simulink model "parafoil_CMA"  (R2024a)
settings: Solver=ode4  StartTime=0.0  StopTime=500  FixedStep=2e-2  RelTol=1e-3
undefined symbols (not defined in the file): F, height_action, MIL, Severe
libraries: aerolibwind2 x1
settings Model: Creator=Long  LastModifiedBy=Yang
settings SolverCC: AlgebraicLoopSolver=TrustRegion
settings DebuggingCC: UnconnectedInputMsg=warning  UnconnectedOutputMsg=warning  UnconnectedLineMsg=warning
settings ModelReferenceCC: EnableRefExpFcnMdlSchedulingChecks=on
settings SFSimCC: CustomCodeUndefinedFunction=UseInterfaceOnly
settings RTWCC: GPUComputeCapability=3.5

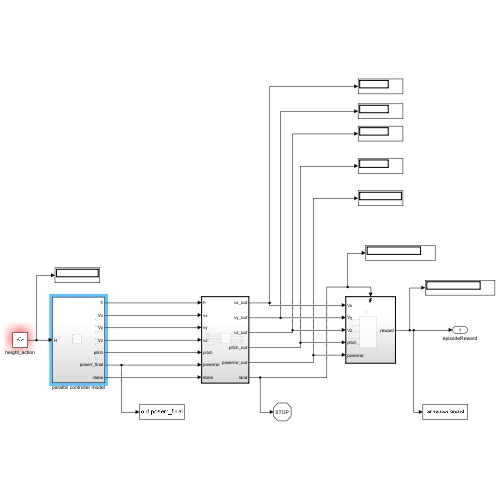
[thumbnail: Simulink's stored preview of the top-level diagram]
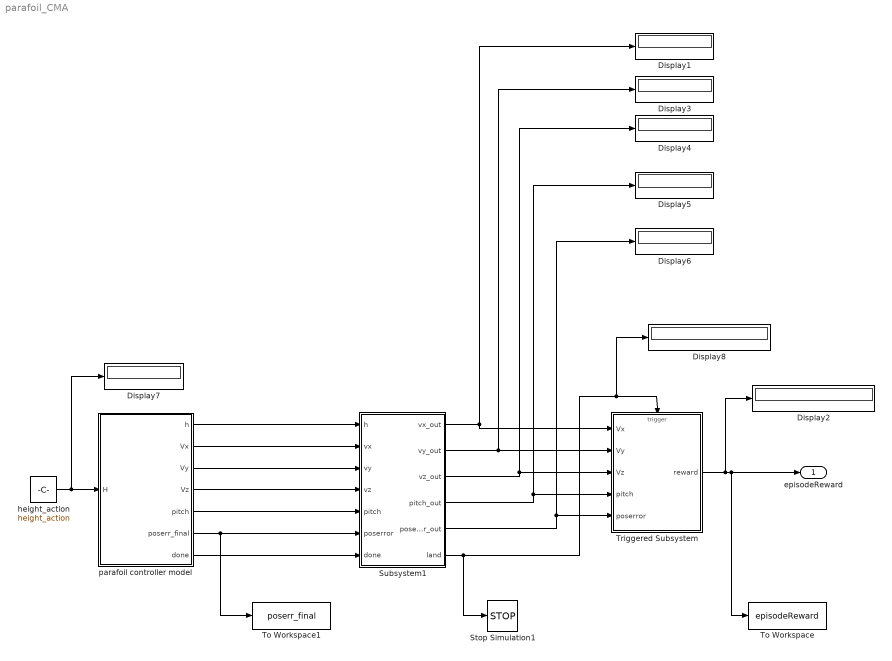
== system parafoil_CMA ==
  Display{1..8} (8 alike) : Display
  Stop Simulation1 : Stop
  Subsystem1 : Subsystem  TreatAsAtomicUnit=on  SystemSampleTime=0.02
  To Workspace : ToWorkspace  VariableName=episodeReward  SampleTime=-1
      settings: MaxDataPoints=1
  To Workspace1 : ToWorkspace  VariableName=poserr_final  SampleTime=-1
      settings: MaxDataPoints=1
  Triggered Subsystem : Subsystem  TreatAsAtomicUnit=on
  height_action : Constant  Value=height_action
  parafoil controller model : Subsystem
  episodeReward : Outport
  wires:
  height_action/1 -> Display7/1, parafoil controller model/1(H)
  Triggered Subsystem/1(reward) -> Display2/1, To Workspace/1, episodeReward/1
  Subsystem1/4(pitch_out) -> Triggered Subsystem/4(pitch), Display5/1
  Subsystem1/2(vy_out) -> Triggered Subsystem/2(Vy), Display3/1
  Subsystem1/5(poserror_out) -> Triggered Subsystem/5(poserror), Display6/1
  Subsystem1/1(vx_out) -> Triggered Subsystem/1(Vx), Display1/1
  Subsystem1/3(vz_out) -> Triggered Subsystem/3(Vz), Display4/1
  parafoil controller model/1(h) -> Subsystem1/1(h)
  parafoil controller model/2(Vx) -> Subsystem1/2(vx)
  parafoil controller model/3(Vy) -> Subsystem1/3(vy)
  parafoil controller model/4(Vz) -> Subsystem1/4(vz)
  parafoil controller model/5(pitch) -> Subsystem1/5(pitch)
  Subsystem1/6(land) -> Stop Simulation1/1, Display8/1, Triggered Subsystem/Trigger
  parafoil controller model/7(done) -> Subsystem1/7(done)
  parafoil controller model/6(poserr_final) -> To Workspace1/1, Subsystem1/6(poserror)

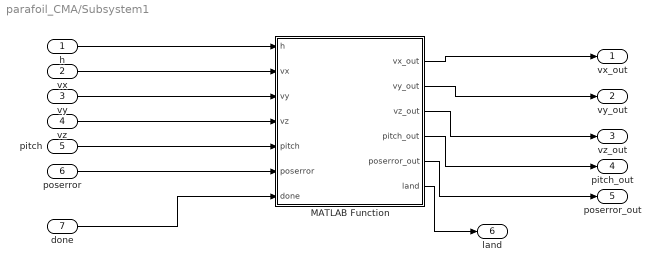
== system parafoil_CMA/Subsystem1 ==
  h : Inport
  vx : Inport  Port=2
  vy : Inport  Port=3
  vz : Inport  Port=4
  pitch : Inport  Port=5
  poserror : Inport  Port=6
  done : Inport  Port=7
  MATLAB Function : MATLAB Function  TreatAsAtomicUnit=on
  vx_out : Outport
  vy_out : Outport  Port=2
  vz_out : Outport  Port=3
  pitch_out : Outport  Port=4
  poserror_out : Outport  Port=5
  land : Outport  Port=6
  wires:
  MATLAB Function/5(poserror_out) -> poserror_out/1
  vx/1 -> MATLAB Function/2(vx)
  MATLAB Function/3(vz_out) -> vz_out/1
  pitch/1 -> MATLAB Function/5(pitch)
  MATLAB Function/1(vx_out) -> vx_out/1
  MATLAB Function/4(pitch_out) -> pitch_out/1
  poserror/1 -> MATLAB Function/6(poserror)
  MATLAB Function/2(vy_out) -> vy_out/1
  vy/1 -> MATLAB Function/3(vy)
  h/1 -> MATLAB Function/1(h)
  vz/1 -> MATLAB Function/4(vz)
  MATLAB Function/6(land) -> land/1
  done/1 -> MATLAB Function/7(done)

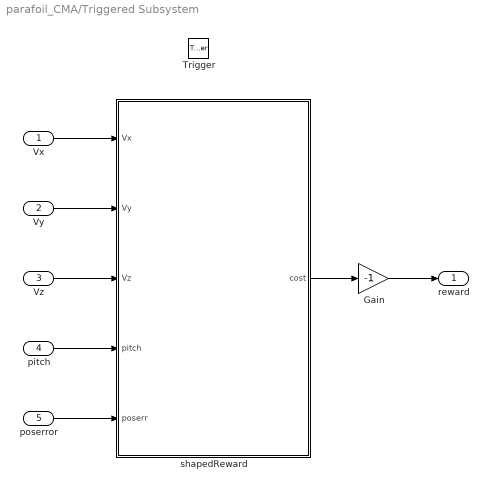
== system parafoil_CMA/Triggered Subsystem ==
  Vx : Inport
  Vy : Inport  Port=2
  Vz : Inport  Port=3
  pitch : Inport  Port=4
  poserror : Inport  Port=5
  Trigger : TriggerPort  VariantControl=(inherit)
  Gain : Gain  Gain=-1
  shapedReward : MATLAB Function  TreatAsAtomicUnit=on
  reward : Outport  VectorParamsAs1DForOutWhenUnconnected=off
  wires:
  pitch/1 -> shapedReward/4(pitch)
  Vy/1 -> shapedReward/2(Vy)
  Vx/1 -> shapedReward/1(Vx)
  poserror/1 -> shapedReward/5(poserr)
  shapedReward/1(cost) -> Gain/1
  Vz/1 -> shapedReward/3(Vz)
  Gain/1 -> reward/1

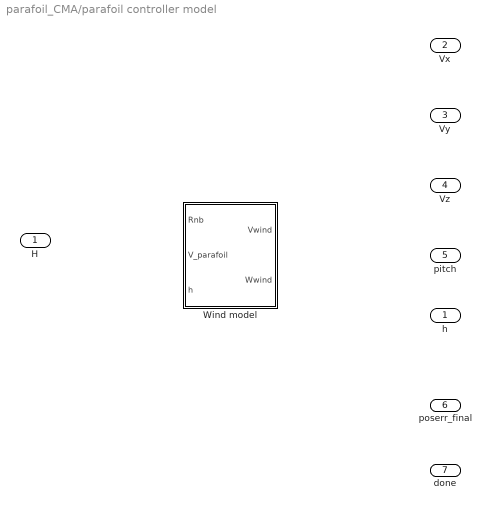
== system parafoil_CMA/parafoil controller model ==
  H : Inport
  Wind model : Subsystem
  h : Outport
  Vx : Outport  Port=2
  Vy : Outport  Port=3
  Vz : Outport  Port=4
  pitch : Outport  Port=5
  poserr_final : Outport  Port=6
  done : Outport  Port=7

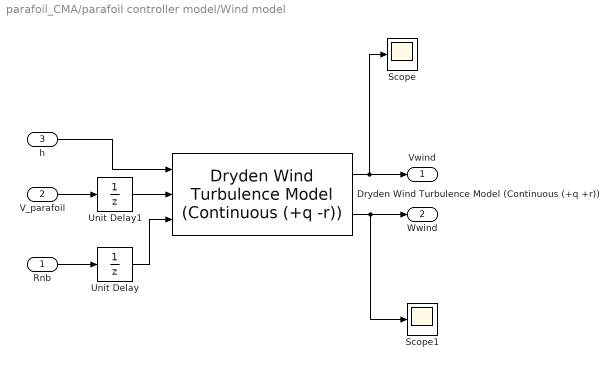
== system parafoil_CMA/parafoil controller model/Wind model ==
  Rnb : Inport
  V_parafoil : Inport  Port=2
  h : Inport  Port=3
  Dryden Wind Turbulence Model (Continuous (+q +r)) : aerolibwind2/Dryden Wind Turbulence Model  (Continuous (+q -r))  units=Metric (MKS)  spec=MIL-F-8785C  model=Continuous Dryden (+q +r)  W20=5  Wdeg=0  TurbProb=10^-5 - Severe  L_high=175  Wingspan=11.18  ts=0.2  Seed=[23341 23342 23343 23344]  T_on=on
      settings: LibrarySourceBlock=|
      | aerolibwind2/Dryden Wind Turbulence Model
      | (Continuous (+q +r))
  Scope : Scope
  Scope1 : Scope
  Unit Delay : UnitDelay  InitialCondition=eye(3)  SampleTime=-1  HasFrameUpgradeWarning=on
  Unit Delay1 : UnitDelay  InitialCondition=1.802  SampleTime=-1  HasFrameUpgradeWarning=on
  Vwind : Outport
  Wwind : Outport  Port=2
  wires:
  h/1 -> Dryden Wind Turbulence Model (Continuous (+q +r))/1
  V_parafoil/1 -> Unit Delay1/1
  Rnb/1 -> Unit Delay/1
  Dryden Wind Turbulence Model (Continuous (+q +r))/1 -> Vwind/1, Scope/1
  Dryden Wind Turbulence Model (Continuous (+q +r))/2 -> Wwind/1, Scope1/1
  Unit Delay/1 -> Dryden Wind Turbulence Model (Continuous (+q +r))/3
  Unit Delay1/1 -> Dryden Wind Turbulence Model (Continuous (+q +r))/2

== matlab function parafoil_CMA/Subsystem1/MATLAB Function ==
  data: h input; vx_out output; vx input; vy input; vz input; pitch input; vy_out output; vz_out output; pitch_out output; poserror input; poserror_out output; land output; done input
function [vx_out, vy_out, vz_out, pitch_out, poserror_out,land] = saveAtZero(h, vx, vy, vz, pitch, poserror, done)
% 简易版：落地前透传；首次 h<=0.01 锁存；之后保持
persistent latched data
if isempty(latched)
    latched = false;
    data    = [vx, vy, vz, pitch, poserror];
end

% 默认输出
land = 0;

if ~latched
    if done == 1
        data    = [vx, vy, vz, pitch, poserror];
        latched = true;
        land=1;
    else
        data = [vx, vy, vz, pitch, poserror];   % 透传
    end
end

vx_out = data(1); vy_out = data(2); vz_out = data(3);
pitch_out = data(4); poserror_out = data(5);
end

== matlab function parafoil_CMA/Triggered Subsystem/shapedReward ==
  data: Vx input; cost output; Vy input; Vz input; pitch input; poserr input
function cost = objective_parafoil(Vx,Vy,Vz,pitch,poserr)
% CMA-ES目标函数：返回单个标量cost，越小越好

% -------- 权重设置 --------
w_pos   = 1.0;    % 位置误差最重要
w_vh    = 2.0;    % 水平速度
w_vz    = 5.0;    % 垂直速度
w_theta = 1.0;    % 姿态角

% -------- 计算派生量 --------
vh = hypot(Vx,Vy);   % 水平速度

% -------- 基础代价 --------
cost = w_pos  * (poserr)^2 ...      % 落点误差（L1）
     + w_vh   * (vh^2) ...           % 水平动能相关项
     + w_vz   * (Vz^2) ...           % 垂直动能相关项（冲击主导）
     + w_theta*50* abs(pitch);           % 姿态平方


% -------- 硬约束（超限直接大惩罚，仍然简洁） --------
pos_max   = 10;              % m
vz_max    = 10;             % m/s
vh_max    = 15;             % m/s
pitch_max = deg2rad(45);    % rad
BIG_M     = 1e3;

% -------- 安全罚分（硬约束） --------
if abs(poserr) > pos_max || vh > vh_max || abs(Vz) > vz_max || abs(pitch) > pitch_max
    cost = cost + BIG_M;   % 超限直接大惩罚
end

end
